simulink model "Sim_sistema_fisico_ordine3"  (R2020a)
settings: Solver=FixedStepAuto  StartTime=0.0  StopTime=StopTime  FixedStep=1/fs  MaxStep=1/fs  MinStep=1/fs  RelTol=1e-3
undefined symbols (not defined in the file): C, K, M
libraries: fl_lib x18, nesl_utility x6
settings Model: Creator=matteo  LastModifiedBy=matteo

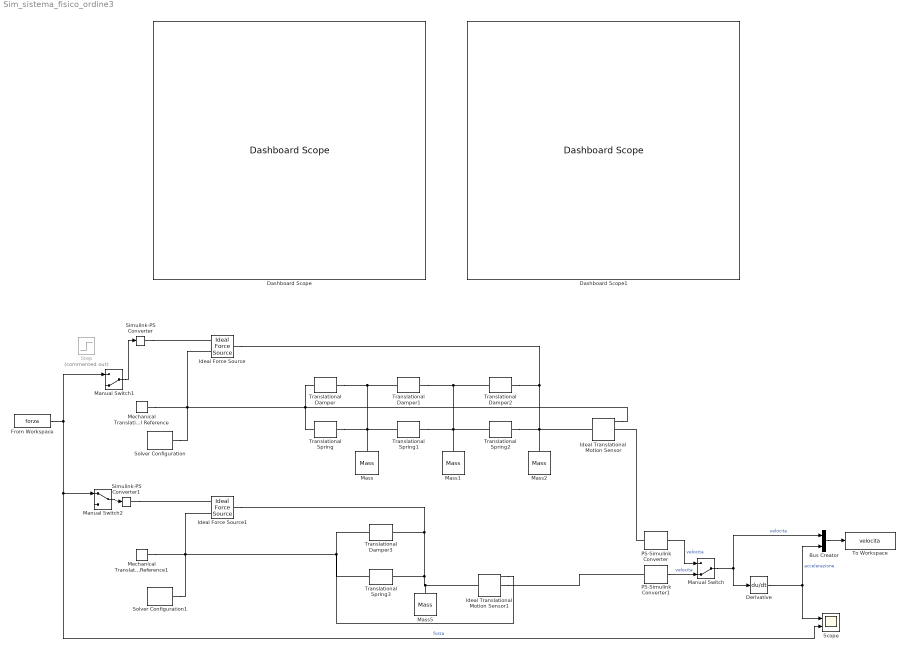
== system Sim_sistema_fisico_ordine3 ==
  Bus Creator : BusCreator  Inputs=2
  Dashboard Scope : DashboardScope
  Dashboard Scope1 : DashboardScope
  Derivative : Derivative
  From Workspace : FromWorkspace  VariableName=forza
  Ideal Force Source : fl_lib/Mechanical/Mechanical Sources/Ideal Force Source
  Ideal Force Source1 : fl_lib/Mechanical/Mechanical Sources/Ideal Force Source
  Ideal Translational Motion Sensor : fl_lib/Mechanical/Mechanical Sensors/Ideal Translational Motion Sensor  offset=0 m
  Ideal Translational Motion Sensor1 : fl_lib/Mechanical/Mechanical Sensors/Ideal Translational Motion Sensor  offset=0 m
  Manual Switch : ManualSwitch  CurrentSetting=0
  Manual Switch1 : ManualSwitch  CurrentSetting=0
  Manual Switch2 : ManualSwitch
  Mass : fl_lib/Mechanical/Translational Elements/Mass  mass=M(3) kg  v_specify=off  v_priority=High  v=0 m/s  v_nominal_specify=off  v_nominal_unit=m/s  v_nominal_value=1  f_specify=off  f_priority=None  f=0 N  f_nominal_specify=off  f_nominal_unit=N  f_nominal_value=1
  Mass1 : fl_lib/Mechanical/Translational Elements/Mass  mass=M(2) kg  v_specify=off  v_priority=High  v=0 m/s  v_nominal_specify=off  v_nominal_unit=m/s  v_nominal_value=1  f_specify=off  f_priority=None  f=0 N  f_nominal_specify=off  f_nominal_unit=N  f_nominal_value=1
  Mass2 : fl_lib/Mechanical/Translational Elements/Mass  mass=M(1) kg  v_specify=off  v_priority=High  v=0 m/s  v_nominal_specify=off  v_nominal_unit=m/s  v_nominal_value=1  f_specify=off  f_priority=None  f=0 N  f_nominal_specify=off  f_nominal_unit=N  f_nominal_value=1
  Mass5 : fl_lib/Mechanical/Translational Elements/Mass  mass=M(1) kg  v_specify=off  v_priority=High  v=0 m/s  v_nominal_specify=off  v_nominal_unit=m/s  v_nominal_value=1  f_specify=off  f_priority=None  f=0 N  f_nominal_specify=off  f_nominal_unit=N  f_nominal_value=1
  Mechanical Translational Reference : fl_lib/Mechanical/Translational Elements/Mechanical Translational Reference
  Mechanical Translational Reference1 : fl_lib/Mechanical/Translational Elements/Mechanical Translational Reference
  PS-Simulink Converter : nesl_utility/PS-Simulink Converter  PhysicalDomain=network_engine_domain  SubClassName=ps_output  LeftPortType=input  RightPortType=output  PseudoPeriodic=off  Frequencies=[]  Unit=inherit  AffineConversion=off
  PS-Simulink Converter1 : nesl_utility/PS-Simulink Converter  PhysicalDomain=network_engine_domain  SubClassName=ps_output  LeftPortType=input  RightPortType=output  PseudoPeriodic=off  Frequencies=[]  Unit=inherit  AffineConversion=off
  Scope : Scope  NumInputPorts=2
  Simulink-PS Converter : nesl_utility/Simulink-PS Converter  PhysicalDomain=network_engine_domain  SubClassName=ps_input  LeftPortType=input  RightPortType=output  PseudoPeriodic=off  Frequencies=[]  NoiseDistribution=none  NoiseParameters=[]  Unit=1  AffineConversion=off  FilteringAndDerivatives=provide  SimscapeFilterOrder=1  InputFilterTimeConstant=0.001  UdotUserProvided=0
  Simulink-PS Converter1 : nesl_utility/Simulink-PS Converter  PhysicalDomain=network_engine_domain  SubClassName=ps_input  LeftPortType=input  RightPortType=output  PseudoPeriodic=off  Frequencies=[]  NoiseDistribution=none  NoiseParameters=[]  Unit=1  AffineConversion=off  FilteringAndDerivatives=provide  SimscapeFilterOrder=1  InputFilterTimeConstant=0.001  UdotUserProvided=0
  Solver Configuration : nesl_utility/Solver Configuration  PhysicalDomain=network_engine_domain  SubClassName=solver  LeftPortType=input  RightPortType=generic  Tones=[]  Harmonics=[]  SimulateNoise=off  Profile=off  UseLocalSampling=off  EnableSwitchedLinearOptims=on  FrequencyDomain=off  UseCCode=off  RelTol=0.001  AbsTol=1e-06  MinStep=1e-09  ToWorkspace=off  RevertToSquareIcSolve=off  NumHomotopyIterations=100  PhasorMode=off  PhasorModeNumHarmonics=1  DoDC=off  ResidualTolerance=1e-09  UseLocalSolver=off  LocalSolverChoice=NE_BACKWARD_EULER_ADVANCER  LocalSolverSampleTime=0.001  DoFixedCost=off  MaxNonlinIter=3  MaxModeIter=2  LinearAlgebra=auto  EquationFormulation=NE_TIME_EF  DelaysMemoryBudget=1024  AutomaticFiltering=on  FilteringTimeConstant=0.001  PartitionStorageMethod=AS_NEEDED  PartitionMemoryBudget=1024  PartitionMethod=ROBUST
  Solver Configuration1 : nesl_utility/Solver Configuration  PhysicalDomain=network_engine_domain  SubClassName=solver  LeftPortType=input  RightPortType=generic  Tones=[]  Harmonics=[]  SimulateNoise=off  Profile=off  UseLocalSampling=off  EnableSwitchedLinearOptims=on  FrequencyDomain=off  UseCCode=off  RelTol=0.001  AbsTol=1e-06  MinStep=1e-09  ToWorkspace=off  RevertToSquareIcSolve=off  NumHomotopyIterations=100  PhasorMode=off  PhasorModeNumHarmonics=1  DoDC=off  ResidualTolerance=1e-09  UseLocalSolver=off  LocalSolverChoice=NE_BACKWARD_EULER_ADVANCER  LocalSolverSampleTime=0.001  DoFixedCost=off  MaxNonlinIter=3  MaxModeIter=2  LinearAlgebra=auto  EquationFormulation=NE_TIME_EF  DelaysMemoryBudget=1024  AutomaticFiltering=on  FilteringTimeConstant=0.001  PartitionStorageMethod=AS_NEEDED  PartitionMemoryBudget=1024  PartitionMethod=ROBUST
  Step : Step  Commented=on  SampleTime=0
  To Workspace : ToWorkspace  VariableName=velocita  SaveFormat=Timeseries  SampleTime=-1
  Translational Damper : fl_lib/Mechanical/Translational Elements/Translational Damper  D=C(3) N/(m/s)  v_specify=off  v_priority=None  v=0 m/s  v_nominal_specify=off  v_nominal_unit=m/s  v_nominal_value=1  f_specify=off  f_priority=None  f=0 N  f_nominal_specify=off  f_nominal_unit=N  f_nominal_value=1
  Translational Damper1 : fl_lib/Mechanical/Translational Elements/Translational Damper  D=C(2) N/(m/s)  v_specify=off  v_priority=None  v=0 m/s  v_nominal_specify=off  v_nominal_unit=m/s  v_nominal_value=1  f_specify=off  f_priority=None  f=0 N  f_nominal_specify=off  f_nominal_unit=N  f_nominal_value=1
  Translational Damper2 : fl_lib/Mechanical/Translational Elements/Translational Damper  D=C(1) N/(m/s)  v_specify=off  v_priority=None  v=0 m/s  v_nominal_specify=off  v_nominal_unit=m/s  v_nominal_value=1  f_specify=off  f_priority=None  f=0 N  f_nominal_specify=off  f_nominal_unit=N  f_nominal_value=1
  Translational Damper3 : fl_lib/Mechanical/Translational Elements/Translational Damper  D=C(2) N/(m/s)  v_specify=off  v_priority=None  v=0 m/s  v_nominal_specify=off  v_nominal_unit=m/s  v_nominal_value=1  f_specify=off  f_priority=None  f=0 N  f_nominal_specify=off  f_nominal_unit=N  f_nominal_value=1
  Translational Spring : fl_lib/Mechanical/Translational Elements/Translational Spring  spr_rate=K(3) N/m  v_specify=off  v_priority=None  v=0 m/s  v_nominal_specify=off  v_nominal_unit=m/s  v_nominal_value=1  f_specify=off  f_priority=None  f=0 N  f_nominal_specify=off  f_nominal_unit=N  f_nominal_value=1  x_specify=off  x_priority=High  x=0 m  x_nominal_specify=off  x_nominal_unit=m  x_nominal_value=1
  Translational Spring1 : fl_lib/Mechanical/Translational Elements/Translational Spring  spr_rate=K(2) N/m  v_specify=off  v_priority=None  v=0 m/s  v_nominal_specify=off  v_nominal_unit=m/s  v_nominal_value=1  f_specify=off  f_priority=None  f=0 N  f_nominal_specify=off  f_nominal_unit=N  f_nominal_value=1  x_specify=off  x_priority=High  x=0 m  x_nominal_specify=off  x_nominal_unit=m  x_nominal_value=1
  Translational Spring2 : fl_lib/Mechanical/Translational Elements/Translational Spring  spr_rate=K(1) N/m  v_specify=off  v_priority=None  v=0 m/s  v_nominal_specify=off  v_nominal_unit=m/s  v_nominal_value=1  f_specify=off  f_priority=None  f=0 N  f_nominal_specify=off  f_nominal_unit=N  f_nominal_value=1  x_specify=off  x_priority=High  x=0 m  x_nominal_specify=off  x_nominal_unit=m  x_nominal_value=1
  Translational Spring3 : fl_lib/Mechanical/Translational Elements/Translational Spring  spr_rate=K(2) N/m  v_specify=off  v_priority=None  v=0 m/s  v_nominal_specify=off  v_nominal_unit=m/s  v_nominal_value=1  f_specify=off  f_priority=None  f=0 N  f_nominal_specify=off  f_nominal_unit=N  f_nominal_value=1  x_specify=off  x_priority=High  x=0 m  x_nominal_specify=off  x_nominal_unit=m  x_nominal_value=1
  wires:
  PS-Simulink Converter/1 -> Manual Switch/1  "velocita"
  From Workspace/1 -> Scope/2, Manual Switch2/1, Manual Switch1/1  "forza"
  Derivative/1 -> Scope/1, Bus Creator/2  "accelerazione"
  Bus Creator/1 -> To Workspace/1
  PS-Simulink Converter1/1 -> Manual Switch/2  "velocita"
  Manual Switch/1 -> Bus Creator/1, Derivative/1  "velocita"
  Manual Switch1/1 -> Simulink-PS Converter/1
  Manual Switch2/1 -> Simulink-PS Converter1/1
  connections:
  Translational Damper/RConn1 -- Translational Damper1/LConn1 -- Translational Spring1/LConn1 -- Translational Spring/RConn1 -- Mass/LConn1
  Translational Damper1/RConn1 -- Translational Damper2/LConn1 -- Translational Spring2/LConn1 -- Translational Spring1/RConn1 -- Mass1/LConn1
  Simulink-PS Converter/RConn1 -- Ideal Force Source/RConn1
  PS-Simulink Converter/LConn1 -- Ideal Translational Motion Sensor/RConn2
  Translational Damper2/RConn1 -- Ideal Translational Motion Sensor/LConn1 -- Mass2/LConn1 -- Translational Spring2/RConn1 -- Ideal Force Source/LConn1
  Ideal Translational Motion Sensor1/RConn2 -- PS-Simulink Converter1/LConn1
  Ideal Translational Motion Sensor/RConn1 -- Ideal Force Source/RConn2 -- Solver Configuration/RConn1 -- Mechanical Translational Reference/LConn1 -- Translational Damper/LConn1 -- Translational Spring/LConn1
  Ideal Translational Motion Sensor1/LConn1 -- Translational Spring3/RConn1 -- Ideal Force Source1/LConn1 -- Translational Damper3/RConn1 -- Mass5/LConn1
  Translational Damper3/LConn1 -- Ideal Translational Motion Sensor1/RConn1 -- Translational Spring3/LConn1 -- Ideal Force Source1/RConn2 -- Mechanical Translational Reference1/LConn1 -- Solver Configuration1/RConn1
  Simulink-PS Converter1/RConn1 -- Ideal Force Source1/RConn1
